simulink model "nonLinearSusMod"  (R2023a)
settings: Solver=VariableStepAuto  StartTime=0.0  StopTime=10.0  RelTol=1e-3
settings Model: Creator=user  LastModifiedBy=Abdulrahman Hamdy

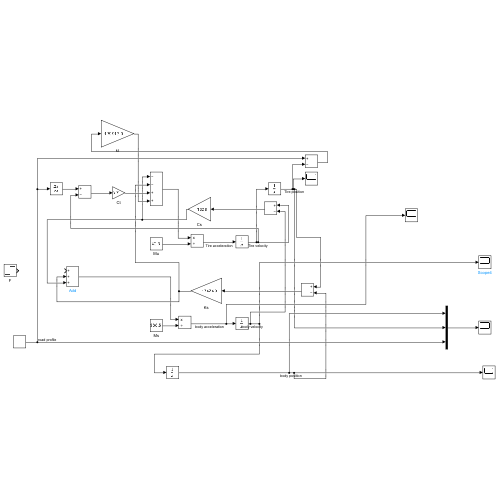
[thumbnail: Simulink's stored preview of the top-level diagram]
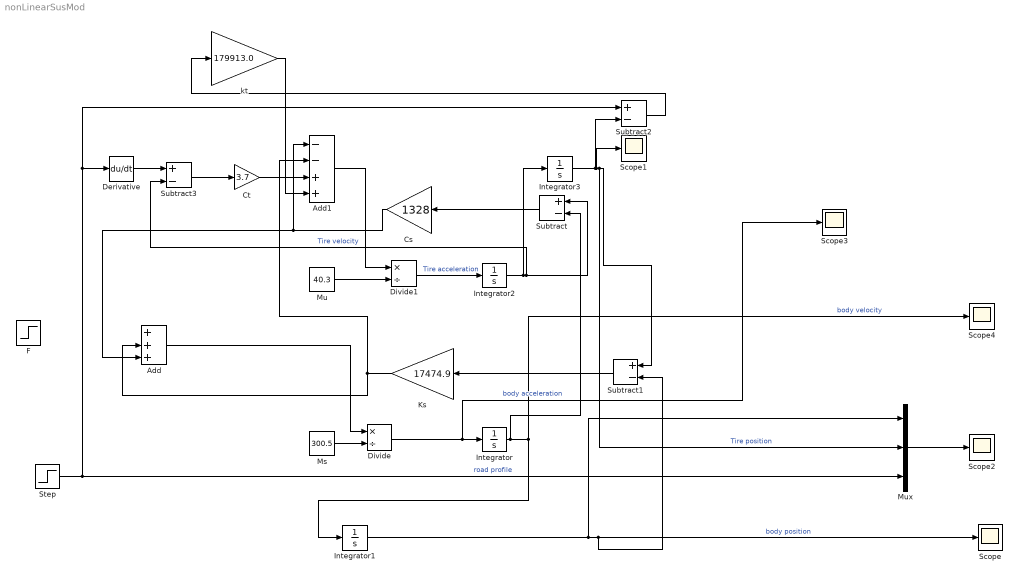
== system nonLinearSusMod ==
  Add : Sum  Inputs=+++
  Add1 : Sum  Inputs=--++
  Cs : Gain  Gain=1328
  Ct : Gain  Gain=3.7
  Derivative : Derivative
  Divide : Product  Inputs=*/
  Divide1 : Product  Inputs=*/
  F : Step  Time=0  After=0  SampleTime=0
  Integrator{,1..3} (4 alike) : Integrator
  Ks : Gain  Gain=17474.9
  Ms : Constant  Value=300.5
  Mu : Constant  Value=40.3
  Mux : Mux  Inputs=3
  Scope{,1..4} (5 alike) : Scope
  Step : Step  SampleTime=0
  Subtract{,1..3} (4 alike) : Sum  Inputs=+-
  kt : Gain  Gain=179913.0
  wires:
  Step/1 -> Derivative/1, Subtract2/1, Mux/3  "road profile"
  Derivative/1 -> Subtract3/1
  Subtract3/1 -> Ct/1
  kt/1 -> Add1/4
  Add1/1 -> Divide1/1
  Ct/1 -> Add1/3
  Mu/1 -> Divide1/2
  Add/1 -> Divide/1
  Ms/1 -> Divide/2
  Cs/1 -> Add1/1, Add/3
  Ks/1 -> Add1/2, Add/2
  Divide1/1 -> Integrator2/1  "Tire acceleration"
  Divide/1 -> Scope3/1, Integrator/1  "body acceleration"
  Integrator2/1 -> Subtract/1, Subtract3/2, Integrator3/1  "Tire velocity"
  Integrator/1 -> Integrator1/1, Scope4/1, Subtract/2  "body velocity"
  Subtract/1 -> Cs/1
  Integrator3/1 -> Subtract1/1, Mux/2, Scope1/1, Subtract2/2  "Tire position"
  Integrator1/1 -> Scope/1, Subtract1/2, Mux/1  "body position"
  Subtract1/1 -> Ks/1
  Subtract2/1 -> kt/1
  Mux/1 -> Scope2/1
